simulink library "Lib_PF_ActiveConvEffDC2AC_TMATS"  (R2017a)
settings: Solver=ode45  StartTime=0.0  StopTime=10.0  RelTol=1e-3  EnableMultiTasking=on
Description:
  | Thomas Modules
settings Model: Creator=jwchapm2  LastModifiedBy=glthoma1
settings DataIOCC: LimitDataPoints=on  SaveFormat=Array
settings OptimizationCC: ExpressionDepthLimit=2147483647  LifeSpan=inf
settings DebuggingCC: UnderspecifiedInitializationDetection=Classic  MergeDetectMultiDrivingBlocksExec=none  SolverPrmCheckMsg=warning  StateNameClashWarn=warning  SFUnexpectedBacktrackingDiag=warning  SFNoUnconditionalDefaultTransitionDiag=warning  SFExecutionAtInitializationDiag=none
settings HardwareCC: ProdBitPerPointer=32  ProdBitPerSizeT=32  ProdBitPerPtrDiffT=32  ProdLargestAtomicFloat=None  ProdIntDivRoundTo=Undefined  ProdEndianess=Unspecified  ProdWordSize=32  ProdHWDeviceType=32-bit Generic
settings ModelReferenceCC: PropagateSignalLabelsOutOfModel=off
settings GRTTargetCC: TargetLangStandard=C89/C90 (ANSI)  GeneratePreprocessorConditionals=Disable all
settings ConfigComp: CovMetricSettings=dw  CovHtmlReporting=on  CovSaveCumulativeToWorkspaceVar=on  CovSaveSingleToWorkspaceVar=on  CovExternalEMLEnable=off

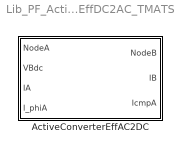
== system Lib_PF_ActiveConvEffDC2AC_TMATS ==
  ActiveConverterEffAC2DC : Subsystem  mask{EffInEN_M=off, Eff_M=98, BlkNm_M=double(gcb)}
      mask prompts: EffInEN_M "EffInEN_M - Externally Defined Efficiency"; Eff_M "Eff_M - Converter Efficiency"; BlkNm_M "Block name as double for simulink output"
      mask init:
      | %Manage Inputs
      | if EffInEN_M == 1
      |     if strcmp(get_param([BlkNm_M '/Eff'],'BlockType'),'Constant')
      |         MSK_ReplaceBlock_TMATS([BlkNm_M '/Eff'],'built-in/Inport');
      |     end
      |     set_param([BlkNm_M '/Eff'],'Port',num2str(5));
      | elseif EffInEN_M == 0
      |     if strcmp(get_param([BlkNm_M '/Eff'],'BlockType'),'Inport')
      |         MSK_ReplaceBlock_TMATS([BlkNm_M '/Eff'],'built-in/Constant');
      |         set_param([BlkNm_M '/Eff'],'Value','Eff_M');
      |     end
      | end
      mask Callback EffInEN_M: MSK_SEC_Enables_TMATS('EffInEN_M',2,'dis')
      mask Display:
      | fprintf('AC : DC')
      | port_label('input',1,'VA')
      | port_label('input',2,'VBdc')
      | port_label('input',3,'IAg')
      | port_label('input',4,'I_phiAg')
      | if EffInEN_M == 1
      | port_label('input',5,'Eff')
      | end
      | port_label('output',1,'VB')
      | port_label('output',2,'IB')
      | port_label('output',3,'IcA')

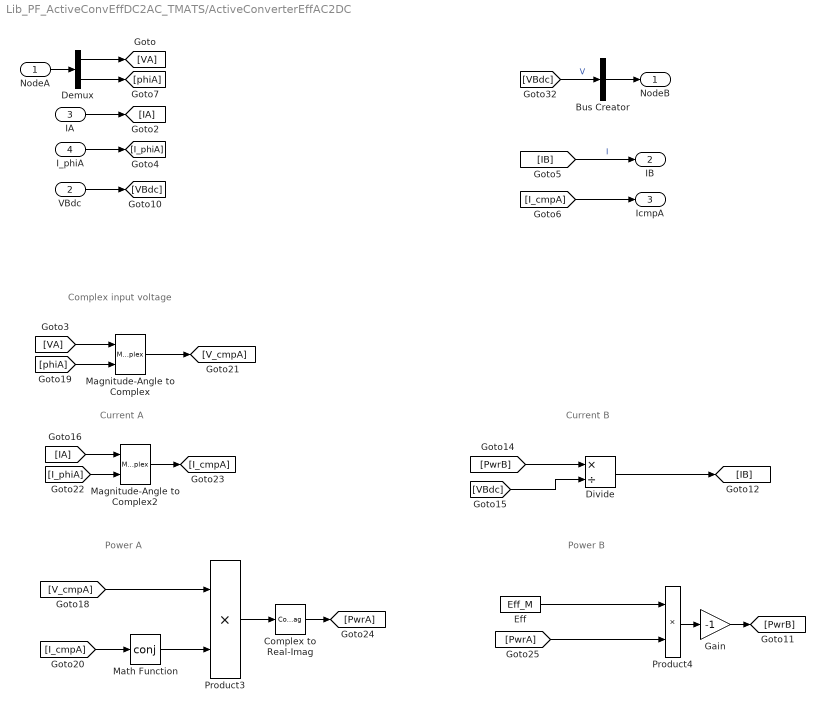
== system Lib_PF_ActiveConvEffDC2AC_TMATS/ActiveConverterEffAC2DC ==
  note: Current A
  note: Power B
  note: Complex input voltage
  note: Power A
  note: Current B
  NodeA : Inport
  VBdc : Inport  Port=2
  IA : Inport  Port=3
  I_phiA : Inport  Port=4
  Bus Creator : BusCreator  Inputs=1
  Complex to Real-Imag : ComplexToRealImag  Output=Real
  Demux : Demux  Outputs=2
  Divide : Product  Inputs=*/
  Eff : Constant  Value=Eff_M
  Gain : Gain  Gain=-1
  Magnitude-Angle to Complex : MagnitudeAngleToComplex
  Magnitude-Angle to Complex2 : MagnitudeAngleToComplex
  Math Function : Math  Operator=conj  SaturateOnIntegerOverflow=on
  Product3 : Product
  Product4 : Product
  NodeB : Outport
  IB : Outport  Port=2
  IcmpA : Outport  Port=3
  wires:
  [PwrA] -> Product4/2
  [PwrB] -> Divide/1
  Magnitude-Angle to Complex/1 -> [V_cmpA]
  [VBdc] -> Divide/2
  I_phiA/1 -> [I_phiA]
  [phiA] -> Magnitude-Angle to Complex/2
  VBdc/1 -> [VBdc]
  [I_phiA] -> Magnitude-Angle to Complex2/2
  [IA] -> Magnitude-Angle to Complex2/1
  Eff/1 -> Product4/1
  Product3/1 -> Complex to Real-Imag/1
  Complex to Real-Imag/1 -> [PwrA]
  [V_cmpA] -> Product3/1
  [I_cmpA] -> IcmpA/1
  [VBdc] -> Bus Creator/1  "V"
  IA/1 -> [IA]
  Math Function/1 -> Product3/2
  Demux/2 -> [phiA]
  Bus Creator/1 -> NodeB/1
  [VA] -> Magnitude-Angle to Complex/1
  Gain/1 -> [PwrB]
  Divide/1 -> [IB]
  [IB] -> IB/1  "I"
  [I_cmpA] -> Math Function/1
  NodeA/1 -> Demux/1
  Product4/1 -> Gain/1
  Demux/1 -> [VA]
  Magnitude-Angle to Complex2/1 -> [I_cmpA]
